simulink model "fullModelStart_jd"  (R2016b)
settings: Solver=ode45  StartTime=0.0  StopTime=10.0  RelTol=1e-3  EnableMultiTasking=on
PreLoadFcn:
  | sensorChapter2;
  | logicChapter3;
  | controllerChapter4;
  | throttleChapter5;
undefined symbols (not defined in the file): degConv, J, Ki, Kp, sigbuilder_block, Ts
settings Model: Creator=jrivitus  LastModifiedBy=training-ah
settings SolverCC: MaxConsecutiveZCs=25
settings DataIOCC: LimitDataPoints=on  SaveFormat=Array
settings OptimizationCC: ExpressionDepthLimit=2147483647  InitFltsAndDblsToZero=on  LifeSpan=inf
settings DebuggingCC: UnderspecifiedInitializationDetection=Classic  MergeDetectMultiDrivingBlocksExec=none  ParameterPrecisionLossMsg=none  FcnCallInpInsideContextMsg=warning  AllowSymbolicDim=off  StateNameClashWarn=warning  SFUnexpectedBacktrackingDiag=warning  SFNoUnconditionalDefaultTransitionDiag=warning  SFExecutionAtInitializationDiag=none
settings HardwareCC: ProdBitPerPointer=32  ProdBitPerSizeT=32  ProdBitPerPtrDiffT=32  ProdLargestAtomicFloat=None  ProdIntDivRoundTo=Undefined  ProdEndianess=Unspecified  ProdWordSize=32  ProdHWDeviceType=32-bit Generic
settings ModelReferenceCC: PropagateSignalLabelsOutOfModel=off
settings GRTTargetCC: TargetLangStandard=C89/C90 (ANSI)  GeneratePreprocessorConditionals=Disable all  CombineOutputUpdateFcns=off  GRTInterface=on
settings ConfigComp: CovMetricSettings=dw  CovHtmlReporting=on  CovSaveCumulativeToWorkspaceVar=on  CovSaveSingleToWorkspaceVar=on  CovExternalEMLEnable=off  CovSFcnEnable=off

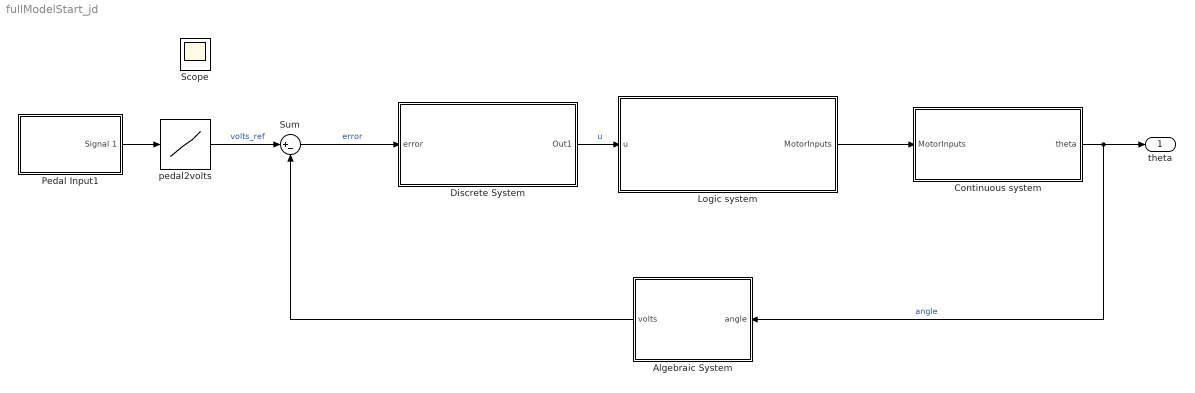
== system fullModelStart_jd ==
  Algebraic System : Subsystem
      mask Display: disp('Sensor');
  Continuous system : Subsystem
      mask Display: disp('Throttle');
  Discrete System : Subsystem
      mask Display: disp('PI Controller');
  Logic system : Subsystem
      mask Display: disp('PWM Conversion');
  Pedal Input1 : Subsystem  Tag=STV Subsys  LoadFcn=sigbuilder_block('load');  StartFcn=sigbuilder_block('start');  StopFcn=sigbuilder_block('stop');  ClipboardFcn=sigbuilder_block('clipboard');  mask(Sigbuilder block){tuvar=[0:10]}
      mask help: Sigbuilder GUI
      mask init:
      | if ~strcmp(get_param(bdroot(gcbh),'SimulationStatus'),'stopped') tuvar = sigbuilder_block('maskInit'); end
      settings: AttributesFormatString=0 - Pedal not pressed\n1 - Pedal fully pressed  CopyFcn=sigbuilder_block('copy');  DeleteFcn=sigbuilder_block('delete');  ModelCloseFcn=sigbuilder_block('modelClose');  PreSaveFcn=sigbuilder_block('preSave');  PauseFcn=sigbuilder_block('pause')  ContinueFcn=sigbuilder_block('continue')  NameChangeFcn=sigbuilder_block('namechange');  OpenFcn=sigbuilder_block('open',[437.6 199.2 550.4 400 ]);  CloseFcn=sigbuilder_block('close');
      mask Display: plot(0,0,100,100,[10,10,40,40,10],[80,20,20,80,80],[40,10],[50,50], [40,27,10],[65,72,56],[40,25,25,10],[28,28,43,43]);
  Sum : Sum  Inputs=|+-
  pedal2volts : Lookup_n-D  NumberOfTableDimensions=1  BreakpointsForDimension1=[0 1]  Table=[0.5 4.5]  RndMeth=Simplest  InputSameDT=on
  theta : Outport
  Scope : Scope
  wires:
  Pedal Input1/1(Signal 1) -> pedal2volts/1
  pedal2volts/1 -> Sum/1  "volts_ref"
  Sum/1 -> Discrete System/1(error)  "error"
  Continuous system/1(theta) -> Algebraic System/1(angle), theta/1  "angle"
  Algebraic System/1(volts) -> Sum/2
  Discrete System/1(Out1) -> Logic system/1(u)  "u"
  Logic system/1(MotorInputs) -> Continuous system/1(MotorInputs)

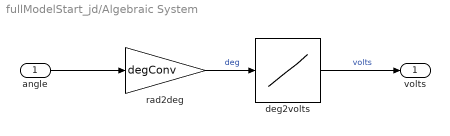
== system fullModelStart_jd/Algebraic System ==
  angle : Inport
  deg2volts : Lookup_n-D  NumberOfTableDimensions=1  BreakpointsForDimension1=[0 90]  Table=[0.5 4.5]  RndMeth=Simplest  InputSameDT=on
  rad2deg : Gain  Gain=degConv  SaturateOnIntegerOverflow=on  OutDataTypeStr=Inherit: Same as input  ParamDataTypeStr=Inherit: Same as input
  volts : Outport
  wires:
  deg2volts/1 -> volts/1  "volts"
  angle/1 -> rad2deg/1
  rad2deg/1 -> deg2volts/1  "deg"

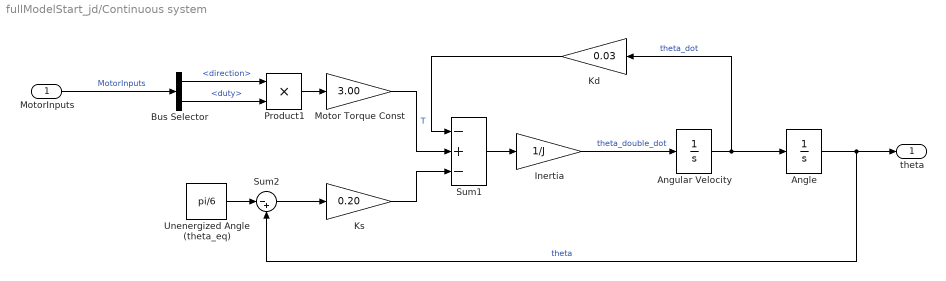
== system fullModelStart_jd/Continuous system ==
  MotorInputs : Inport
  Angle : Integrator  InitialCondition=pi/6  LimitOutput=on  UpperSaturationLimit=pi/2  LowerSaturationLimit=0
      settings: AttributesFormatString=Initial condition: %<InitialCondition>\n%<LowerSaturationLimit> <= theta <= %<UpperSaturationLimit>
  Angular Velocity : Integrator
      settings: AttributesFormatString=Initial condition: %<InitialCondition>
  Bus Selector : BusSelector  OutputSignals=direction,duty
  Inertia : Gain  Gain=1/J  SaturateOnIntegerOverflow=on  OutDataTypeStr=Inherit: Same as input  ParamDataTypeStr=Inherit: Same as input
  Kd : Gain  Gain=0.03  SaturateOnIntegerOverflow=on  OutDataTypeStr=Inherit: Same as input  ParamDataTypeStr=Inherit: Same as input
  Ks : Gain  Gain=0.20  SaturateOnIntegerOverflow=on  OutDataTypeStr=Inherit: Same as input  ParamDataTypeStr=Inherit: Same as input
  Motor Torque Const : Gain  Gain=3.00  SaturateOnIntegerOverflow=on  OutDataTypeStr=Inherit: Same as input  ParamDataTypeStr=Inherit: Same as input
  Product1 : Product  SaturateOnIntegerOverflow=on  OutDataTypeStr=Inherit: Same as first input
  Sum1 : Sum  Inputs=-+-  SaturateOnIntegerOverflow=on
  Sum2 : Sum  Inputs=|-+  SaturateOnIntegerOverflow=on
  Unenergized Angle (theta_eq) : Constant  Value=pi/6
  theta : Outport
  wires:
  Sum2/1 -> Ks/1
  Sum1/1 -> Inertia/1
  Angle/1 -> theta/1, Sum2/2  "theta"
  Kd/1 -> Sum1/1
  Unenergized Angle (theta_eq)/1 -> Sum2/1
  Angular Velocity/1 -> Kd/1, Angle/1  "theta_dot"
  Motor Torque Const/1 -> Sum1/2  "T"
  Ks/1 -> Sum1/3
  Product1/1 -> Motor Torque Const/1
  Inertia/1 -> Angular Velocity/1  "theta_double_dot"
  Bus Selector/1 -> Product1/1  "<direction>"
  Bus Selector/2 -> Product1/2  "<duty>"
  MotorInputs/1 -> Bus Selector/1  "MotorInputs"

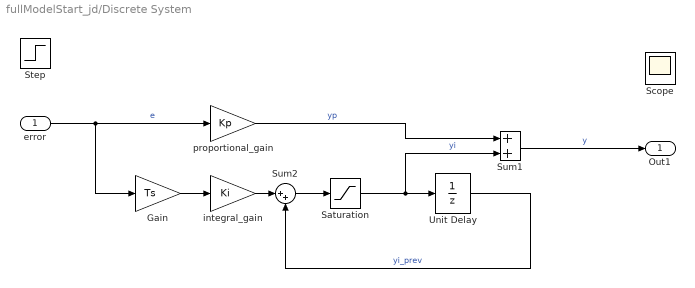
== system fullModelStart_jd/Discrete System ==
  error : Inport
  Gain : Gain  Gain=Ts  SaturateOnIntegerOverflow=on  OutDataTypeStr=Inherit: Same as input  ParamDataTypeStr=Inherit: Same as input
  Saturation : Saturate  UpperLimit=1  LowerLimit=-1
      settings: AttributesFormatString=Max: %<UpperLimit>\nMin: %<LowerLimit>
  Scope : Scope
  Step : Step  SampleTime=Ts
      settings: AttributesFormatString=Sample time = %<SampleTime>
  Sum1 : Sum  SaturateOnIntegerOverflow=on  InputSameDT=on  OutDataTypeStr=Inherit: Same as first input
  Sum2 : Sum  Inputs=|++  SaturateOnIntegerOverflow=on  InputSameDT=on  OutDataTypeStr=Inherit: Same as first input
  Unit Delay : UnitDelay  SampleTime=Ts
      settings: AttributesFormatString=yi0 = %<X0>\nSample time = %<SampleTime>
  integral_gain : Gain  Gain=Ki  SaturateOnIntegerOverflow=on  OutDataTypeStr=Inherit: Same as input  ParamDataTypeStr=Inherit: Same as input
  proportional_gain : Gain  Gain=Kp  SaturateOnIntegerOverflow=on  OutDataTypeStr=Inherit: Same as input  ParamDataTypeStr=Inherit: Same as input
  Out1 : Outport
  wires:
  Sum2/1 -> Saturation/1
  Sum1/1 -> Out1/1  "y"
  Unit Delay/1 -> Sum2/2  "yi_prev"
  Saturation/1 -> Sum1/2, Unit Delay/1  "yi"
  proportional_gain/1 -> Sum1/1  "yp"
  integral_gain/1 -> Sum2/1
  error/1 -> Gain/1, proportional_gain/1  "e"
  Gain/1 -> integral_gain/1

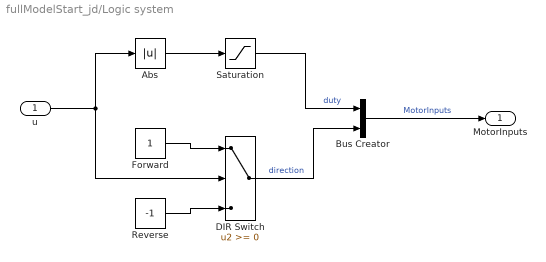
== system fullModelStart_jd/Logic system ==
  u : Inport
  Abs : Abs
  Bus Creator : BusCreator  Inputs=2
  DIR Switch : Switch
      settings: AttributesFormatString=Criteria: %<Criteria>\nThreshold: %<Threshold>
  Forward : Constant  OutDataTypeStr=double
  Reverse : Constant  Value=-1  OutDataTypeStr=double
  Saturation : Saturate  UpperLimit=1  LowerLimit=0
      settings: AttributesFormatString=%<LowerLimit> < duty < %<UpperLimit>
  MotorInputs : Outport
  wires:
  Abs/1 -> Saturation/1
  Reverse/1 -> DIR Switch/3
  DIR Switch/1 -> Bus Creator/2  "direction"
  Saturation/1 -> Bus Creator/1  "duty"
  Forward/1 -> DIR Switch/1
  u/1 -> Abs/1, DIR Switch/2
  Bus Creator/1 -> MotorInputs/1  "MotorInputs"

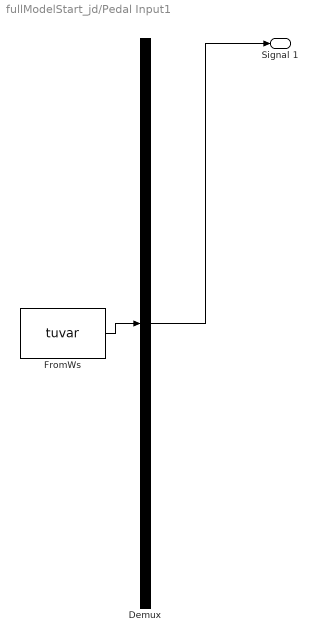
== system fullModelStart_jd/Pedal Input1 ==
  Demux : Demux  Tag=STV Demux  Outputs=1
  FromWs : FromWorkspace  Tag=STV FromWs  VariableName=tuvar  SampleTime=0
      SigBuilderData=|
      | common.afterFinalStr = 'Extrapolate'
      | common.sampleTime = 0
      | dataSet.timeRange = [0 10]
      | dataSet.name = 'Group 1'
      | sbobj.Groups.Name = 'Group 1'
      | sbobj.Groups.Signals.Name = 'Signal 1'
      | sbobj.Groups.Signals.XData = [0 2 2 6 6 10]
      | sbobj.Groups.Signals.YData = [0 0 0.8 0.8 0.2 0.2]
  Signal 1 : Outport  Tag=STV Outport
  wires:
  FromWs/1 -> Demux/1
  Demux/1 -> Signal 1/1
